simulink model "standalone_plant_test"  (R2026a)
settings: Solver=VariableStepAuto  StopTime=20
undefined symbols (not defined in the file or in its folder): EnumF16FailureType
libraries: simulink x1
settings Model: Creator=Edison Altamirano  LastModifiedBy=Edison Altamirano

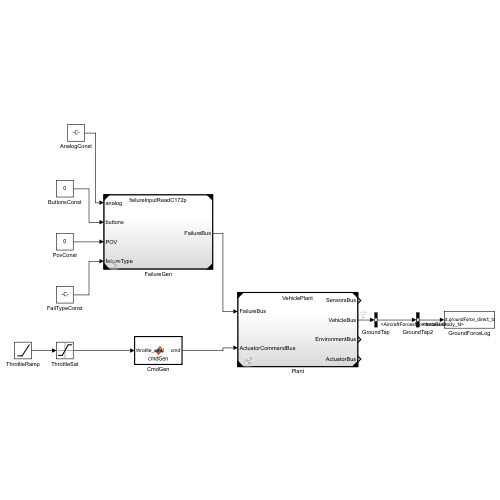
[thumbnail: Simulink's stored preview of the top-level diagram]
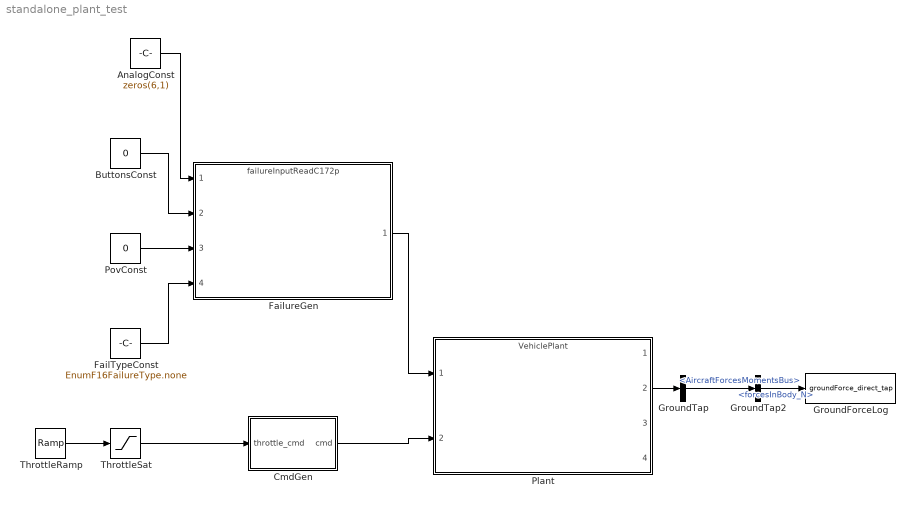
== system standalone_plant_test ==
  AnalogConst : Constant  Value=zeros(6,1)
  ButtonsConst : Constant  Value=0  OutDataTypeStr=uint32
  CmdGen : MATLAB Function  TreatAsAtomicUnit=on
  FailTypeConst : Constant  Value=EnumF16FailureType.none  OutDataTypeStr=Enum: EnumF16FailureType
  FailureGen : ModelReference  ModelNameDialog=failureInputReadC172p.slx  ModelReferenceVersion=1.18
  GroundForceLog : ToWorkspace  VariableName=groundForce_direct_tap  SaveFormat=Structure With Time
  GroundTap : BusSelector  OutputSignals=AircraftForcesMomentsBus
  GroundTap2 : BusSelector  OutputSignals=forcesInBody_N
  Plant : ModelReference  ModelNameDialog=VehiclePlant.slx  ModelReferenceVersion=5.12
  PovConst : Constant  Value=0
  ThrottleRamp : simulink/Sources/Ramp  slope=0.5  start=0  InitialOutput=0
  ThrottleSat : Saturate  UpperLimit=1  LowerLimit=0
  wires:
  AnalogConst/1 -> FailureGen/1
  ButtonsConst/1 -> FailureGen/2
  PovConst/1 -> FailureGen/3
  FailTypeConst/1 -> FailureGen/4
  FailureGen/1 -> Plant/1
  ThrottleRamp/1 -> ThrottleSat/1
  ThrottleSat/1 -> CmdGen/1(throttle_cmd)
  CmdGen/1(cmd) -> Plant/2
  Plant/2 -> GroundTap/1
  GroundTap/1 -> GroundTap2/1  "<AircraftForcesMomentsBus>"
  GroundTap2/1 -> GroundForceLog/1  "<forcesInBody_N>"

== matlab function standalone_plant_test/CmdGen ==
  data: throttle_cmd input; cmd output Bus: ActuatorCommandBus
function cmd = cmdGen(throttle_cmd)
%#codegen
cmd.controllerArmed = 1;
cmd.ServosCommandBus.ServosCommandFixedwingPlaneBus.cmdAileron_nd = 0;
cmd.ServosCommandBus.ServosCommandFixedwingPlaneBus.cmdElevator_nd = 0;
cmd.ServosCommandBus.ServosCommandFixedwingPlaneBus.cmdRudder_nd = 0;
cmd.EngineCommandBus.cmdThrottle_unit = throttle_cmd;
end
